simulink model "Bit_test"  (R2020b)
settings: Solver=VariableStepAuto  StartTime=0.0  StopTime=10.0  RelTol=1e-3
settings Model: Creator=Triphase_Setup  LastModifiedBy=Triphase_Setup

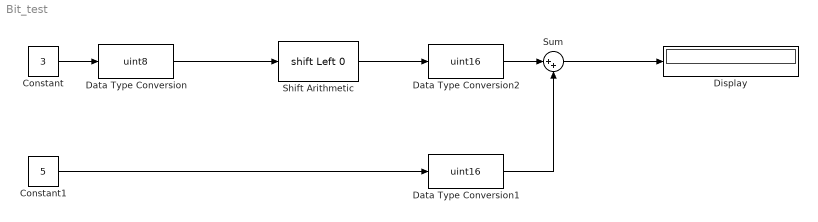
== system Bit_test ==
  Constant : Constant  Value=3
  Constant1 : Constant  Value=5
  Data Type Conversion : DataTypeConversion  OutDataTypeStr=uint8
  Data Type Conversion1 : DataTypeConversion  OutDataTypeStr=uint16
  Data Type Conversion2 : DataTypeConversion  OutDataTypeStr=uint16
  Display : Display
  Shift Arithmetic : ArithShift  BinPtShiftNumber=8  BitShiftDirection=Left
  Sum : Sum  Inputs=|++
  wires:
  Constant/1 -> Data Type Conversion/1
  Constant1/1 -> Data Type Conversion1/1
  Data Type Conversion/1 -> Shift Arithmetic/1
  Shift Arithmetic/1 -> Data Type Conversion2/1
  Data Type Conversion2/1 -> Sum/1
  Data Type Conversion1/1 -> Sum/2
  Sum/1 -> Display/1
